simulink model "tqdtqr_rebuild_V3"  (R2021b)
settings: Solver=VariableStepAuto  StartTime=0.0  StopTime=10.0  RelTol=1e-3
undefined symbols (not defined in the file): ATQD_AfterTqMinGain_X_Deg, ATQD_APSCreepBaseTqD_X_kph, ATQD_APSCreepBaseTqD_Y_Deg, ATQD_APSCreepBaseTqR_X_kph, ATQD_APSCreepBaseTqR_Y_Deg, ATQD_APSCreepIterm_X_kph, ATQD_APSCreepIterm_Y_kph, ATQD_APSCreepPterm_X_kph, ATQD_APSCreepPterm_Y_kph, ATQD_APSDecReq_X_kph, ATQD_APSDecReq_Y_mps2, ATQD_APSDecReqCMD_X_kph, ATQD_APSDecReqTs_X_pct, ATQD_APSDecTimeGain_X_Deg, ATQD_APSDecTimeGain_Y_s, ATQD_APSReqLowSpd_X_Deg, ATQD_AutoHoldReleaseBPS_X_Deg, ATQD_AWDLoadTrqnsGain_X_kg, ATQD_AWDLoadTrqnsGain_Y_pct, ATQD_BOSEnBPSPosn_X_kph, ATQD_BOSMap_X_rpm, ATQD_BOSMap_Y_pct, ATQD_CreepBaseTqD_X_kph, ATQD_CreepBaseTqD_Y_Deg, ATQD_CreepBaseTqR_X_kph, ATQD_CreepBaseTqR_Y_Deg, ATQD_CreepBPSDisPosn_X_Deg, ATQD_CreepBPSDisPosnR_X_Deg, ATQD_CreepBPSEnPosn_X_Deg, ATQD_CreepBPSEnPosnR_X_Deg, ATQD_CreepDeltaTq_X_kph, ATQD_CreepIterm_X_kph, ATQD_CreepIterm_Y_kph, ATQD_CreepItermMaxLimit_X_pct, ATQD_CreepPreloadTime_X_kph, ATQD_CreepPreloadTq_X_kph, ATQD_CreepPreloadTq_Y_s, ATQD_CreepProtTq_X_Deg, ATQD_CreepPterm_X_kph, ATQD_CreepPterm_Y_kph, ATQD_CreepRrTqSpRat_X_rpm, ATQD_CreepRrTqSpRat_Y_Nm, ATQD_CreepTargetSpdD_X_pct, ATQD_CreepTargetSpdR_X_pct, ATQD_CreepUpLimitTq_X_rpm, ATQD_DecIneOPDHoldEnDelay_X_Deg, ATQD_DecIneOPDHoldEnDelay_Y_bar, ATQD_ECOTqMapD_X_rpm, ATQD_ECOTqMapD_Y_pct, ATQD_EMTqMapD_X_rpm, ATQD_EMTqMapD_Y_pct, ATQD_EOPDTqMapDCon_X_rpm, ATQD_EOPDTqMapDCon_Y_Deg, ATQD_EstInitVehWeight_X_c, ATQD_FAfterTqCMDGain_X_rpm, ATQD_FAfterTqCMDGain_Y_pct, ATQD_ForceLowSpd_X_Deg, ATQD_ForcePLimitSpd_X_Deg, ATQD_FrLossMAPLowV_X_rpm, ATQD_FrLossMAPLowV_Y_Nm ... (+949)
libraries: simulink x235, hcu_lib x208, tqr x63, tqd x6
(part 12 of 37)

== system tqdtqr_rebuild_V3/Input_Convert/Signal function/MCU Damping Disable Judgement ==
  note: Front / Rear final damping disable flag with vehicle type
  note: Damping disable requested by APS / vehicle speed
  note: Front/Rear MCU damping disable flag
  BSCPIn_outputs : Inport
  BSignalConvert_outputs : Inport  Port=2
  AND2 : Logic  Operator=OR  AllPortsSameDT=off  OutDataTypeStr=boolean
  AND9 : Logic  Operator=OR  AllPortsSameDT=off  OutDataTypeStr=boolean
  Bus Selector : BusSelector  OutputSignals=VVMC_ADASActive_flg,VINP_FrRBCActive_flg,VINP_FrntAxlTrqReqBrk_Nm,VVMC_ACCRequiredAccel_mps2,VINP_RrRBCActive_flg,VINP_RearAxlTrqReqBrk_Nm,VINP_VehSpeed_kph,VTQD_ActAPSPosn_pct,VPMM_DrivetrainSelect_enum
  Bus Selector1 : BusSelector  OutputSignals=VTQD_SCPFrEDURealTMTq_Nm,VTQD_SCPRrEDURealTMTq_Nm
  Constant24 : Constant  Value=KTQD_MCUDmEnFrBrkTq_Nm
  Constant25 : Constant  Value=KTQD_MCUDmEnAccCMD_mps2
  Constant27 : Constant  Value=KTQD_MCUDmEnRrBrkTq_Nm
  Constant40 : Constant  Value=KTQD_ActvDmpDisabAPSPosn_pct  OutDataTypeStr=Inherit: Inherit via back propagation
  Constant41 : Constant  Value=KTQD_ActvDmpDisabVehSpd_kph  OutDataTypeStr=Inherit: Inherit via back propagation
  Constant44 : Constant  Value=KTQD_MCUDmEnAccCMD_mps2
  Constant48 : Constant  Value=ENUM_DRIVETRAIN_FWD
  Constant49 : Constant  Value=ENUM_DRIVETRAIN_AWD
  Constant59 : Constant  Value=ENUM_DRIVETRAIN_RWD
  Constant60 : Constant  Value=ENUM_DRIVETRAIN_AWD
  Constant61 : Constant  Value=FALSE
  Constant62 : Constant  Value=FALSE
  Constant63 : Constant  Value=KTQD_RrDmpDisabReq_flg_ovrdval  OutDataTypeStr=Inherit: Inherit via back propagation
  Constant64 : Constant  Value=KTQD_FrDmpDisabReq_flg_ovrdval  OutDataTypeStr=Inherit: Inherit via back propagation
  Constant65 : Constant  Value=KTQD_MCUDmEnRrBrkTq_Nm
  Constant67 : Constant  Value=KTQD_FrDmpDisabReq_flg_ovrdflg  OutDataTypeStr=Inherit: Inherit via back propagation
  Constant68 : Constant  Value=KTQD_RrDmpDisabReq_flg_ovrdflg  OutDataTypeStr=Inherit: Inherit via back propagation
  Constant9 : Constant  Value=KTQD_MCUDmEnFrBrkTq_Nm
  Data Type Conversion : DataTypeConversion  OutDataTypeStr=boolean
  Data Type Conversion1 : DataTypeConversion  OutDataTypeStr=boolean
  Equal{17..19,23} (4 alike) : RelationalOperator  Operator===  OutDataTypeStr=boolean  RndMeth=Simplest
  Equal{24..25,27..28} (4 alike) : RelationalOperator  OutDataTypeStr=boolean  RndMeth=Simplest
  Equal26 : RelationalOperator  Operator=>  OutDataTypeStr=boolean  RndMeth=Simplest
  Equal29 : RelationalOperator  Operator=>  OutDataTypeStr=boolean  RndMeth=Simplest
  Less Than : RelationalOperator  Operator=<=  OutDataTypeStr=boolean  RndMeth=Simplest
  Less Than1 : RelationalOperator  Operator=<=  OutDataTypeStr=boolean  RndMeth=Simplest
  LiuzgSwitch{16..17,19..20} (4 alike) : Switch  Criteria=u2 ~= 0
      settings: AttributesFormatString=<%<Criteria>>
  Logical Operator{7,10,12..13,15,17..18} (7 alike) : Logic  AllPortsSameDT=off  OutDataTypeStr=boolean
  Logical Operator11 : Logic  Operator=OR  Inputs=3  AllPortsSameDT=off  OutDataTypeStr=boolean
  Logical Operator14 : Logic  Operator=OR  Inputs=3  AllPortsSameDT=off  OutDataTypeStr=boolean
  Logical Operator16 : Logic  Operator=NOT  AllPortsSameDT=off  OutDataTypeStr=boolean
  Logical Operator19 : Logic  Operator=OR  AllPortsSameDT=off  OutDataTypeStr=boolean
  Logical Operator8 : Logic  Operator=OR  AllPortsSameDT=off  OutDataTypeStr=boolean
  Logical Operator9 : Logic  Operator=NOT  AllPortsSameDT=off  OutDataTypeStr=boolean
  Relay : Relay  OnSwitchValue=KTQD_FrMCUDmDisSpd_kph  OffSwitchValue=KTQD_FrMCUDmEnSpd_kph
      settings: AttributesFormatString=|
      | ON : %<OffSwitchValue>
      | OFF : %<OnSwitchValue>
  Relay1 : Relay  OnSwitchValue=KTQD_RrMCUDmDisSpd_kph  OffSwitchValue=KTQD_RrMCUDmEnSpd_kph
      settings: AttributesFormatString=|
      | ON : %<OffSwitchValue>
      | OFF : %<OnSwitchValue>
  SR_Latch1 : hcu_lib/Basic_Blocks/SR_Latch
  SR_Latch2 : hcu_lib/Basic_Blocks/SR_Latch
  VTQD_FrActvDmpDisabReq_flg : Outport
  VTQD_RrActvDmpDisabReq_flg : Outport  Port=2
  wires:
  [VTQD_ActAPSPosn_pct] -> Less Than/1
  LiuzgSwitch17/1 -> LiuzgSwitch20/3
  [VPMM_DrivetrainSelect_enum] -> Equal17/1
  AND2/1 -> LiuzgSwitch16/2
  Logical Operator8/1 -> LiuzgSwitch17/1
  Equal26/1 -> Logical Operator11/3
  [VINP_VehSpeed_kph] -> Relay1/1
  [VINP_FrntAxlTrqReqBrk_Nm] -> Equal24/1
  Constant59/1 -> Equal17/2
  Less Than/1 -> Logical Operator7/1
  Constant61/1 -> LiuzgSwitch16/3
  LiuzgSwitch20/1 -> [VTQD_RrActvDmpDisabReq_flg]  "VTQD_RrActvDmpDisabReq_flg"
  Relay/1 -> Data Type Conversion/1
  [VVMC_ADASActive_flg] -> Logical Operator15/1
  Data Type Conversion/1 -> Logical Operator17/1  "VTQD_FrMCUDmDisSpd_flg"
  Equal24/1 -> Logical Operator10/1
  LiuzgSwitch19/1 -> [VTQD_FrActvDmpDisabReq_flg]  "VTQD_FrActvDmpDisabReq_flg"
  [VTQD_FrADASRegMCUDmDis_flg] -> Logical Operator19/1
  Constant62/1 -> LiuzgSwitch17/3
  Constant41/1 -> Less Than1/2
  [VTQD_RrADASRegMCUDmDis_flg] -> Logical Operator8/1
  Equal18/1 -> AND2/1
  AND9/1 -> LiuzgSwitch17/2
  Constant64/1 -> LiuzgSwitch19/1
  SR_Latch1/1 -> Logical Operator17/2
  [VINP_FrRBCActive_flg] -> Logical Operator12/2
  Data Type Conversion1/1 -> Logical Operator18/1  "VTQD_RrMCUDmDisSpd_flg"
  Constant9/1 -> Equal24/2
  Constant24/1 -> Equal25/2
  Logical Operator14/1 -> SR_Latch2/2
  Constant67/1 -> LiuzgSwitch19/2
  Less Than1/1 -> Logical Operator7/2
  [VINP_FrRBCActive_flg] -> Logical Operator9/1
  [VTQD_SCPFrEDURealTMTq_Nm] -> Equal25/1
  [VVMC_ACCRequiredAccel_mps2] -> Equal29/1
  [VINP_RrRBCActive_flg] -> Logical Operator16/1
  Logical Operator19/1 -> LiuzgSwitch16/1
  Relay1/1 -> Data Type Conversion1/1
  Equal29/1 -> Logical Operator14/3
  Equal25/1 -> Logical Operator10/2
  Logical Operator12/1 -> SR_Latch1/1
  [VTQD_MCUDmpDisabReq_flg] -> Logical Operator8/2
  Constant68/1 -> LiuzgSwitch20/2
  Constant49/1 -> Equal19/2
  Constant60/1 -> Equal23/2
  Equal23/1 -> AND9/2
  SR_Latch2/1 -> Logical Operator18/2
  [VINP_VehSpeed_kph] -> Relay/1
  Logical Operator10/1 -> Logical Operator11/1
  [VTQD_MCUDmpDisabReq_flg] -> Logical Operator19/2
  [VTQD_SCPRrEDURealTMTq_Nm] -> Equal28/1
  Constant63/1 -> LiuzgSwitch20/1
  Equal28/1 -> Logical Operator13/2
  Constant25/1 -> Equal26/2
  Logical Operator17/1 -> [VTQD_FrADASRegMCUDmDis_flg]  "VTQD_FrADASRegMCUDmDis_flg"
  [VINP_RearAxlTrqReqBrk_Nm] -> Equal27/1
  Constant40/1 -> Less Than/2
  Constant48/1 -> Equal18/2
  Logical Operator7/1 -> [VTQD_MCUDmpDisabReq_flg]  "VTQD_MCUDmpDisabReq_flg"
  Equal19/1 -> AND2/2
  Logical Operator16/1 -> Logical Operator14/2
  [VPMM_DrivetrainSelect_enum] -> Equal19/1
  Equal27/1 -> Logical Operator13/1
  [VVMC_ADASActive_flg] -> Logical Operator12/1
  Logical Operator11/1 -> SR_Latch1/2
  Constant27/1 -> Equal28/2
  Logical Operator13/1 -> Logical Operator14/1
  [VPMM_DrivetrainSelect_enum] -> Equal18/1
  Equal17/1 -> AND9/1
  [VVMC_ACCRequiredAccel_mps2] -> Equal26/1
  Constant65/1 -> Equal27/2
  Logical Operator9/1 -> Logical Operator11/2
  [VPMM_DrivetrainSelect_enum] -> Equal23/1
  Logical Operator18/1 -> [VTQD_RrADASRegMCUDmDis_flg]  "VTQD_RrADASRegMCUDmDis_flg"
  [VINP_VehSpeed_kph] -> Less Than1/1
  Constant44/1 -> Equal29/2
  [VINP_RrRBCActive_flg] -> Logical Operator15/2
  LiuzgSwitch16/1 -> LiuzgSwitch19/3
  Logical Operator15/1 -> SR_Latch2/1
  BSCPIn_outputs/1 -> Bus Selector/1
  Bus Selector/1 -> [VVMC_ADASActive_flg]  "<VVMC_ADASActive_flg>"
  Bus Selector/2 -> [VINP_FrRBCActive_flg]  "<VINP_FrRBCActive_flg>"
  Bus Selector/3 -> [VINP_FrntAxlTrqReqBrk_Nm]  "<VINP_FrntAxlTrqReqBrk_Nm>"
  BSignalConvert_outputs/1 -> Bus Selector1/1
  Bus Selector1/1 -> [VTQD_SCPFrEDURealTMTq_Nm]  "<VTQD_SCPFrEDURealTMTq_Nm>"
  Bus Selector/4 -> [VVMC_ACCRequiredAccel_mps2]  "<VVMC_ACCRequiredAccel_mps2>"
  Bus Selector/5 -> [VINP_RrRBCActive_flg]  "<VINP_RrRBCActive_flg>"
  Bus Selector/6 -> [VINP_RearAxlTrqReqBrk_Nm]  "<VINP_RearAxlTrqReqBrk_Nm>"
  Bus Selector/7 -> [VINP_VehSpeed_kph]  "<VINP_VehSpeed_kph>"
  Bus Selector1/2 -> [VTQD_SCPRrEDURealTMTq_Nm]  "<VTQD_SCPRrEDURealTMTq_Nm>"
  Bus Selector/8 -> [VTQD_ActAPSPosn_pct]  "<VTQD_ActAPSPosn_pct>"
  Bus Selector/9 -> [VPMM_DrivetrainSelect_enum]  "<VPMM_DrivetrainSelect_enum>"
  [VTQD_RrActvDmpDisabReq_flg] -> VTQD_RrActvDmpDisabReq_flg/1
  [VTQD_FrActvDmpDisabReq_flg] -> VTQD_FrActvDmpDisabReq_flg/1

== system tqdtqr_rebuild_V3/Input_Convert/Signal function/New Wheel Slide Rate ==
  note: Get vehicle speed base
  note: Get max and min slide rate
  note: Calculate left front wheel slide rate
  note: Calculate right front wheel slide rate
  note: Calculate right rear wheel slide rate
  note: Compare front rear slide rate percent
  note: Calculate left rear wheel slide rate
  note: Compare left right slide rate percent
  BSCPIn_outputs : Inport
  BMain_outputs : Inport  Port=2
  Abs{,1..7} (8 alike) : Abs
  Add : Sum
  Add{1..4} (4 alike) : Sum  Inputs=+-
  Bus Selector : BusSelector  OutputSignals=task_time_s,VINP_RRRawWhlSpeed_kph,VINP_RFRawWhlSpeed_kph,VINP_LRRawWhlSpeed_kph,VINP_LFRawWhlSpeed_kph,VINP_VehSpeed_kph
  Bus Selector1 : BusSelector  OutputSignals=VTQR_NoABSREDUWhlTqReq_Nm,VTQR_NoABSFEDUWhlTqReq_Nm
  Constant{1,4,6,9,11,15,18,135} (8 alike) : Constant  Value=eps
  Constant{5,10,14,128} (4 alike) : Constant  Value=KTQD_NewSlideRateTs_c
  Constant{2,7,12,16,19} (5 alike) : Constant  Value=ZERO_FLOAT
  Constant{3,8,13,17} (4 alike) : Constant  Value=ONE_PERCENT
  Data Type Conversion{,1..3} (4 alike) : DataTypeConversion  OutDataTypeStr=single
  Delay : Delay  DelayLength=1  InitialCondition=single(0.0)
      settings: AttributesFormatString=%<InitialCondition>
  Delay1 : Delay  DelayLength=1  InitialCondition=single(0.0)
      settings: AttributesFormatString=%<InitialCondition>
  Divide{,1..7} (8 alike) : Product  Inputs=*/
  FirstOrderFilter{,1..3} (4 alike) : hcu_lib/Basic_Blocks/FirstOrderFilter
  Max{,1..3} (4 alike) : MinMax  Function=max  Inputs=2
  Max4 : MinMax  Function=max  Inputs=4
  Max5 : MinMax  Inputs=4
  Min : MinMax  Inputs=5
  Relational Operator{,1..3} (4 alike) : RelationalOperator  Operator=<=  OutDataTypeStr=boolean  RndMeth=Simplest
  Relational Operator{4..7} (4 alike) : RelationalOperator  OutDataTypeStr=boolean  RndMeth=Simplest
  Relational Operator8 : RelationalOperator  Operator=>  OutDataTypeStr=boolean  RndMeth=Simplest
  Switch{,1..8} (9 alike) : Switch  Criteria=u2 ~= 0
      settings: AttributesFormatString=%<Criteria>
  VTQD_MaxWhlSlideRate_pct : Outport
  VTQD_MinWhlSlideRate_pct : Outport  Port=2
  VTQD_LeftSlideRate_pct : Outport  Port=3
  VTQD_RightSlideRate_pct : Outport  Port=4
  VTQD_FrontSlideRate_pct : Outport  Port=5
  VTQD_RearSlideRate_pct : Outport  Port=6
  VTQD_LFSlideRate_pct : Outport  Port=7
  VTQD_LRSlideRate_pct : Outport  Port=8
  VTQD_RFSlideRate_pct : Outport  Port=9
  VTQD_RRSlideRate_pct : Outport  Port=10
  wires:
  BSCPIn_outputs/1 -> Bus Selector/1
  Bus Selector/1 -> [task_time_s]  "<task_time_s>"
  Bus Selector/3 -> [VINP_RFRawWhlSpeed_kph]  "<VINP_RFRawWhlSpeed_kph>"
  Bus Selector/2 -> [VINP_RRRawWhlSpeed_kph]  "<VINP_RRRawWhlSpeed_kph>"
  Bus Selector/6 -> [VINP_VehSpeed_kph]  "<VINP_VehSpeed_kph>"
  Bus Selector/5 -> [VINP_LFRawWhlSpeed_kph]  "<VINP_LFRawWhlSpeed_kph>"
  Bus Selector/4 -> [VINP_LRRawWhlSpeed_kph]  "<VINP_LRRawWhlSpeed_kph>"
  [VTQD_MaxWhlSlideRate_pct] -> VTQD_MaxWhlSlideRate_pct/1
  [VTQD_MinWhlSlideRate_pct] -> VTQD_MinWhlSlideRate_pct/1
  [VTQD_LeftSlideRate_pct] -> VTQD_LeftSlideRate_pct/1
  [VTQD_RightSlideRate_pct] -> VTQD_RightSlideRate_pct/1
  [VTQD_FrontSlideRate_pct] -> VTQD_FrontSlideRate_pct/1
  [VTQD_RearSlideRate_pct] -> VTQD_RearSlideRate_pct/1
  [VTQD_LFSlideRate_pct] -> VTQD_LFSlideRate_pct/1
  [VTQD_LRSlideRate_pct] -> VTQD_LRSlideRate_pct/1
  [VTQD_RFSlideRate_pct] -> VTQD_RFSlideRate_pct/1
  [VTQD_RRSlideRate_pct] -> VTQD_RRSlideRate_pct/1
  Abs3/1 -> Relational Operator5/2
  [VTQR_NoABSFEDUWhlTqReq_Nm] -> Delay/1
  Constant11/1 -> Data Type Conversion/1
  [VTQD_VehSpeed4Cal_kph] -> Max1/1
  Data Type Conversion/1 -> Max2/2
  Constant6/1 -> Data Type Conversion1/1
  Data Type Conversion1/1 -> Max1/2
  Data Type Conversion2/1 -> Max/2
  Abs2/1 -> Relational Operator5/1
  Divide5/1 -> Switch2/3
  Constant15/1 -> Data Type Conversion3/1
  Constant135/1 -> Data Type Conversion2/1
  Data Type Conversion3/1 -> Max3/2
  FirstOrderFilter1/1 -> Divide2/1
  Switch6/1 -> [VTQD_FrontSlideRate_pct]  "VTQD_FrontSlideRate_pct"
  [VTQD_VehSpeed4Cal_kph] -> Add3/2
  Switch/1 -> FirstOrderFilter/1
  Add3/1 -> Divide5/1
  [VTQD_VehSpeed4Cal_kph] -> Max3/1
  [VTQD_VehSpeed4Cal_kph] -> Max2/1
  Max2/1 -> Divide5/2
  [VTQD_LRSlideRate_pct] -> Abs1/1
  [VINP_RRRawWhlSpeed_kph] -> Add4/1
  FirstOrderFilter/1 -> Divide/1
  Abs1/1 -> Relational Operator4/2
  [VTQD_RFSlideRate_pct] -> Max4/3
  Constant1/1 -> Relational Operator/2
  Abs5/1 -> Relational Operator6/2
  Relational Operator/1 -> Switch/2
  [VTQD_VehSpeed4Cal_kph] -> Max/1
  Constant4/1 -> Relational Operator1/2
  [task_time_s] -> FirstOrderFilter3/2
  [VTQD_VehSpeed4Cal_kph] -> Add4/2
  [VTQD_RFSlideRate_pct] -> Switch6/3
  [task_time_s] -> FirstOrderFilter2/2
  [VTQD_RRSlideRate_pct] -> Abs3/1
  Constant5/1 -> FirstOrderFilter1/3
  Add/1 -> Relational Operator8/1
  [VTQD_VehSpeed4Cal_kph] -> Add1/2
  [VTQD_LFSlideRate_pct] -> Switch6/1
  [VINP_VehSpeed_kph] -> Min/5
  FirstOrderFilter3/1 -> Divide6/1
  Abs7/1 -> Relational Operator7/2
  Divide6/1 -> [VTQD_RRSlideRate_pct]  "VTQD_RRSlideRate_pct"
  [VTQR_NoABSREDUWhlTqReq_Nm] -> Delay1/1
  [VINP_VehSpeed_kph] -> Switch8/3
  [VINP_LRRawWhlSpeed_kph] -> Min/2
  Relational Operator5/1 -> Switch5/2
  Abs/1 -> Relational Operator4/1
  [VINP_RRRawWhlSpeed_kph] -> Min/4
  [VTQD_VehSpeed4Cal_kph] -> Relational Operator3/1
  Max5/1 -> [VTQD_MinWhlSlideRate_pct]  "VTQD_MinWhlSlideRate_pct"
  [VINP_LFRawWhlSpeed_kph] -> Min/1
  [VTQD_LFSlideRate_pct] -> Max4/1
  Switch8/1 -> [VTQD_VehSpeed4Cal_kph]  "VTQD_VehSpeed4Cal_kph"
  [VTQD_RRSlideRate_pct] -> Switch5/3
  Add2/1 -> Divide1/1
  Delay/1 -> Add/1
  Divide4/1 -> [VTQD_RFSlideRate_pct]  "VTQD_RFSlideRate_pct"
  [VTQD_VehSpeed4Cal_kph] -> Relational Operator1/1
  Constant19/1 -> Relational Operator8/2
  [VTQD_RFSlideRate_pct] -> Abs5/1
  Relational Operator8/1 -> Switch8/2
  Abs4/1 -> Relational Operator6/1
  [VINP_RFRawWhlSpeed_kph] -> Min/3
  Constant13/1 -> Divide4/2
  Max/1 -> Divide1/2
  [VTQD_LFSlideRate_pct] -> Abs4/1
  Switch4/1 -> [VTQD_LeftSlideRate_pct]  "VTQD_LeftSlideRate_pct"
  Divide3/1 -> Switch1/3
  Constant10/1 -> FirstOrderFilter2/3
  Constant17/1 -> Divide6/2
  Relational Operator1/1 -> Switch1/2
  Relational Operator4/1 -> Switch4/2
  Constant7/1 -> Switch1/1
  [VTQD_LRSlideRate_pct] -> Max4/2
  Divide2/1 -> [VTQD_LRSlideRate_pct]  "VTQD_LRSlideRate_pct"
  Relational Operator2/1 -> Switch2/2
  Min/1 -> Switch8/1
  [VTQD_RFSlideRate_pct] -> Abs2/1
  Max1/1 -> Divide3/2
  [VINP_LRRawWhlSpeed_kph] -> Add1/1
  [VTQD_RFSlideRate_pct] -> Switch5/1
  Max4/1 -> [VTQD_MaxWhlSlideRate_pct]  "VTQD_MaxWhlSlideRate_pct"
  [VTQD_RRSlideRate_pct] -> Max5/4
  Constant128/1 -> FirstOrderFilter/3
  Add4/1 -> Divide7/1
  [VTQD_LFSlideRate_pct] -> Switch4/1
  [VTQD_LRSlideRate_pct] -> Max5/2
  [VTQD_LRSlideRate_pct] -> Switch4/3
  Add1/1 -> Divide3/1
  Constant12/1 -> Switch2/1
  Divide1/1 -> Switch/3
  Constant2/1 -> Switch/1
  [VTQD_VehSpeed4Cal_kph] -> Add2/2
  [VTQD_VehSpeed4Cal_kph] -> Relational Operator/1
  [VTQD_RRSlideRate_pct] -> Abs7/1
  [VTQD_RFSlideRate_pct] -> Max5/3
  [VTQD_RRSlideRate_pct] -> Max4/4
  Constant3/1 -> Divide/2
  [VINP_LFRawWhlSpeed_kph] -> Add2/1
  [task_time_s] -> FirstOrderFilter/2
  [VTQD_VehSpeed4Cal_kph] -> Relational Operator2/1
  [VTQD_LRSlideRate_pct] -> Switch7/1
  Divide7/1 -> Switch3/3
  Max3/1 -> Divide7/2
  Delay1/1 -> Add/2
  Switch7/1 -> [VTQD_RearSlideRate_pct]  "VTQD_RearSlideRate_pct"
  [VTQD_LFSlideRate_pct] -> Max5/1
  Relational Operator3/1 -> Switch3/2
  FirstOrderFilter2/1 -> Divide4/1
  Divide/1 -> [VTQD_LFSlideRate_pct]  "VTQD_LFSlideRate_pct"
  Relational Operator7/1 -> Switch7/2
  Abs6/1 -> Relational Operator7/1
  Constant18/1 -> Relational Operator3/2
  [VTQD_RRSlideRate_pct] -> Switch7/3
  Constant14/1 -> FirstOrderFilter3/3
  [VINP_RFRawWhlSpeed_kph] -> Add3/1
  Constant16/1 -> Switch3/1
  Switch5/1 -> [VTQD_RightSlideRate_pct]  "VTQD_RightSlideRate_pct"
  [task_time_s] -> FirstOrderFilter1/2
  Switch1/1 -> FirstOrderFilter1/1
  Constant9/1 -> Relational Operator2/2
  Constant8/1 -> Divide2/2
  Switch3/1 -> FirstOrderFilter3/1
  [VTQD_LFSlideRate_pct] -> Abs/1
  Relational Operator6/1 -> Switch6/2
  Switch2/1 -> FirstOrderFilter2/1
  [VTQD_LRSlideRate_pct] -> Abs6/1
  BMain_outputs/1 -> Bus Selector1/1
  Bus Selector1/1 -> [VTQR_NoABSREDUWhlTqReq_Nm]  "<VTQR_NoABSREDUWhlTqReq_Nm>"
  Bus Selector1/2 -> [VTQR_NoABSFEDUWhlTqReq_Nm]  "<VTQR_NoABSFEDUWhlTqReq_Nm>"

== system tqdtqr_rebuild_V3/Input_Convert/Signal function/OPD Hold ==
  BSCPIn_outputs : Inport
  BSignalConvert_outputs : Inport  Port=2
  DriverWhlTqDemFunc_outputs : Inport  Port=3
  BMain_outputs : Inport  Port=4
  VTQD_GearActualPosn_enum : Inport  Port=5
  VTQD_ActWhlSkipSta_enum : Inport  Port=6
  VTQD_SkipDirect_enum : Inport  Port=7
  VTQD_ParkRequest_flg : Inport  Port=8
  VTQD_ForceP_flg : Inport  Port=9
  VTQD_EPBCarWashMode_flg : Inport  Port=10
  Bus Selector : BusSelector  OutputSignals=task_time_s,VINP_EPBSta_enum,VVMC_ADASActive_flg,VPMM_PowerSta_enum,VVMC_CruzActive_flg,VVMC_EstSlope_Deg,VINP_FrPTCSActive_flg,VINP_RrPTCSActive_flg,VINP_ESCActive_flg,VINP_ABSActive_flg,VVMC_APSActive_flg,VTQD_ActBPSPosn_pct,VTQD_LimpHomeAct_flg,VVMC_LongAcc_Gps,VTQD_ActAPSPosn_pct,VINP_DrDoorSW_flg,VPMM_DrSeatSta_enum,VTQD_ShifterHandleCmd_enum,VINP_BrkSwSta_flg,VINP_DriverSeatBeltCmd_flg,VINP_MCPressure_bar
  Bus Selector1 : BusSelector  OutputSignals=VTQD_RegenMode_enum,VTQD_VehActSpd_kph,VTQD_LowIdleAccPedal_flg,VTQD_TqTargetShaftSpd_rpm
  Bus Selector2 : BusSelector  OutputSignals=VTQR_NoABSFEDUWhlTqReq_Nm,VTQR_NoABSREDUWhlTqReq_Nm
  Bus Selector3 : BusSelector  OutputSignals=VTQD_PedAccTqEn_flg,VTQD_IVIRockModeEn_flg
  Constant34 : Constant  Value=KTQD_IVICreepOnSW_flg
  Deceleration Calculation : Subsystem
  "OPDHold Request " : Subsystem
  Parking Requeest Backup : Subsystem  AncestorBlock=tqd/TQD/TorqueDemand/TorqueModule/OPD Hold/Parking Requeest Backup
  Release Condition : Subsystem
  System Status : Subsystem
  VTQD_APSStaSys_enum : Outport
  VTQD_APSReq_enum : Outport  Port=2
  VTQD_APSDecReqA_flg : Outport  Port=3
  VTQD_APSDecReq_mps2 : Outport  Port=4
  VTQD_ActParkRequest_flg : Outport  Port=5
  VTQD_APSReqTimer_s : Outport  Port=6
  VTQD_OPDHoldEnRel_flg : Outport  Port=7
  VTQD_OPDHoldAllowPark_flg : Outport  Port=8
  VTQD_OPDHoldLamp_flg : Outport  Port=9
  VTQD_OPDHoldActRelTq_Nm : Outport  Port=10
  VTQD_OPDHoldDelayForP_flg : Outport  Port=11
  VTQD_OPDHoldAlarm_flg : Outport  Port=12
  VTQD_OPDHoldForceEn_flg : Outport  Port=13
  wires:
  [VTQD_ActWhlSkipSta_enum] -> System Status/19(VTQD_ActWhlSkipSta_enum)
  [VTQD_LimpHomeAct_flg] -> System Status/21(VTQD_LimpHomeAct_flg)
  [VTQD_PedAccTqEn_flg] -> System Status/16(VTQD_PedAccTqEn_flg)
  [VTQD_SkipDirect_enum] -> System Status/20(VTQD_SkipDirect_enum)
  [task_time_s] -> Release Condition/6(task_time_s)
  [VTQD_APSDecReqA_flg] -> Deceleration Calculation/5(VTQD_APSDecReqA_flg)
  System Status/2(VTQD_OPDHoldDelayForP_flg) -> [VTQD_OPDHoldDelayForP_flg]
  [VTQD_IVIRockModeEn_flg] -> System Status/18(VTQD_IVIRockModeEn_flg)
  [VINP_ABSActive_flg] -> System Status/14(VINP_ABSActive_flg)
  Parking Requeest Backup/2(VTQD_OPDHoldAllowPark_flg) -> [VTQD_OPDHoldAllowPark_flg]
  Deceleration Calculation/1(VTQD_APSDecReq_mps2) -> [VTQD_APSDecReq_mps2]
  "OPDHold Request "/3(VTQD_APSDecReqA_flg) -> [VTQD_APSDecReqA_flg]
  [task_time_s] -> Deceleration Calculation/7(task_time_s)
  [VVMC_EstSlope_Deg] -> Release Condition/1(VVMC_EstSlope_Deg)
  [task_time_s] -> Parking Requeest Backup/4(task_time_s)
  [VTQD_OPDHoldRgnOn2Off_flg] -> Release Condition/9(VTQD_OPDHoldRgnOn2Off_flg)
  System Status/3(VTQD_OPDHoldRgnOn2Off_flg) -> [VTQD_OPDHoldRgnOn2Off_flg]
  [VTQD_AutoHoldRelease_flg] -> System Status/4(VTQD_AutiHoldRelease_flg)
  [VTQD_LowIdleAccPedal_flg] -> Release Condition/8(VTQD_LowIdleAccPedal_flg)
  [VTQD_AutoHoldRelease_flg] -> Deceleration Calculation/6(VTQD_AutiHoldRelease_flg)
  [VTQD_ParkRequest_flg] -> Parking Requeest Backup/3(VTQD_ParkRequest_flg)
  [VVMC_EstSlope_Deg] -> "OPDHold Request "/5(VVMC_EstSlope_Deg)
  [VTQR_NoABSREDUWhlTqReq_Nm] -> Release Condition/4(VTQR_NoABSREDUWhlTqReq_Nm)
  [VTQR_NoABSFEDUWhlTqReq_Nm] -> Release Condition/3(VTQR_NoABSFEDUWhlTqReq_Nm)
  [VVMC_CruzActive_flg] -> System Status/7(VVMC_CruzActive_flg)
  Parking Requeest Backup/1(VTQD_ActParkRequest_flg) -> [VTQD_ActParkRequest_flg]
  [VINP_EPBSta_enum] -> System Status/2(VINP_EPBSta_enum)
  [VTQD_ActBPSPosn_pct] -> Release Condition/5(VTQD_ActBPSPosn_pct)
  [VTQD_AutoHoldRelease_flg] -> Parking Requeest Backup/5(VTQD_AutiHoldRelease_flg)
  [VTQD_RegenMode_enum] -> System Status/3(VTQD_RegenMode_enum)
  [VTQD_GearActualPosn_enum] -> System Status/1(VTQD_GearActualPosn_enum)
  [VVMC_EstSlope_Deg] -> Deceleration Calculation/4(VVMC_EstSlope_Deg)
  [VTQD_APSReqTimer_s] -> Parking Requeest Backup/2(VTQD_APSReqTimer_s)
  [VTQD_APSReqTimer_s] -> Deceleration Calculation/3(VTQD_APSReqTimer_s)
  [VINP_IVICreepOnSW_flg] -> System Status/17(VINP_IVICreepOnSW_flg)
  [VTQD_VehActSpd_kph] -> Deceleration Calculation/1(VTQD_VehActSpd_kph)
  "OPDHold Request "/1(VTQD_APSReqTimer_s) -> [VTQD_APSReqTimer_s]
  [VTQD_AutoHoldRelease_flg] -> "OPDHold Request "/3(VTQD_AutiHoldRelease_flg)
  [VTQD_ActAPSPosn_pct] -> Deceleration Calculation/8(VTQD_ActAPSPosn_pct)
  System Status/1(VTQD_APSStaSys_enum) -> [VTQD_APSStaSys_enum]
  [VTQD_VehActSpd_kph] -> Release Condition/2(VTQD_VehActSpd_kph)
  [VVMC_ADASActive_flg] -> System Status/5(VVMC_ADASActive_flg)
  Release Condition/2(VTQD_OPDHoldEnRel_flg) -> [VTQD_OPDHoldEnRel_flg]
  [VTQD_VehActSpd_kph] -> System Status/8(VTQD_VehActSpd_kph)
  "OPDHold Request "/2(VTQD_APSReq_enum) -> [VTQD_APSReq_enum]
  [VINP_FrPTCSActive_flg] -> System Status/11(VINP_FrPTCSActive_flg)
  [VINP_ESCActive_flg] -> System Status/13(VINP_ESCActive_flg)
  [VINP_RrPTCSActive_flg] -> System Status/12(VINP_RrPTCSActive_flg)
  Release Condition/3(VTQD_OPDHoldActRelTq_Nm) -> [VTQD_OPDHoldActRelTq_Nm]
  [VTQD_APSReqTimer_s] -> Release Condition/7(VTQD_APSReqTimer_s)
  [VTQD_APSReq_enum] -> Parking Requeest Backup/1(VTQD_APSReq_enum)
  [VVMC_EstSlope_Deg] -> System Status/9(VVMC_EstSlope_Deg)
  [VVMC_LongAcc_Gps] -> Deceleration Calculation/2(VVMC_LongAcc_Gps)
  [task_time_s] -> System Status/10(task_time_s)
  [task_time_s] -> "OPDHold Request "/4(task_time_s)
  [VPMM_PwrSta_enum] -> System Status/6(VPMM_PwrSta_enum)
  Release Condition/1(VTQD_AutoHoldRelease_flg) -> [VTQD_AutoHoldRelease_flg]
  [VTQD_APSStaSys_enum] -> "OPDHold Request "/2(VTQD_APSStaSys_enum)
  [VVMC_APSActive_flg] -> System Status/15(VVMC_APSActive_flg)
  "OPDHold Request "/4(VTQD_OPDHoldLamp_flg) -> [VTQD_OPDHoldLamp_flg]
  [VTQD_VehActSpd_kph] -> "OPDHold Request "/1(VTQD_VehActSpd_kph)
  BSCPIn_outputs/1 -> Bus Selector/1
  BSignalConvert_outputs/1 -> Bus Selector1/1
  Bus Selector/2 -> [VINP_EPBSta_enum]  "<VINP_EPBSta_enum>"
  Bus Selector1/1 -> [VTQD_RegenMode_enum]  "<VTQD_RegenMode_enum>"
  Bus Selector/3 -> [VVMC_ADASActive_flg]  "<VVMC_ADASActive_flg>"
  Bus Selector/4 -> [VPMM_PwrSta_enum]  "<VPMM_PowerSta_enum>"
  Bus Selector/5 -> [VVMC_CruzActive_flg]  "<VVMC_CruzActive_flg>"
  Bus Selector1/2 -> [VTQD_VehActSpd_kph]  "<VTQD_VehActSpd_kph>"
  Bus Selector/6 -> [VVMC_EstSlope_Deg]  "<VVMC_EstSlope_Deg>"
  Bus Selector/1 -> [task_time_s]  "<task_time_s>"
  Bus Selector/7 -> [VINP_FrPTCSActive_flg]  "<VINP_FrPTCSActive_flg>"
  Bus Selector/8 -> [VINP_RrPTCSActive_flg]  "<VINP_RrPTCSActive_flg>"
  Bus Selector/9 -> [VINP_ESCActive_flg]  "<VINP_ESCActive_flg>"
  Bus Selector/10 -> [VINP_ABSActive_flg]  "<VINP_ABSActive_flg>"
  Bus Selector/11 -> [VVMC_APSActive_flg]  "<VVMC_APSActive_flg>"
  DriverWhlTqDemFunc_outputs/1 -> Bus Selector3/1
  Bus Selector3/1 -> [VTQD_PedAccTqEn_flg]  "<VTQD_PedAccTqEn_flg>"
  Constant34/1 -> [VINP_IVICreepOnSW_flg]  "VTQD_IVICreepOnSW_flg"
  Bus Selector3/2 -> [VTQD_IVIRockModeEn_flg]  "<VTQD_IVIRockModeEn_flg>"
  Bus Selector/12 -> [VTQD_ActBPSPosn_pct]  "<VTQD_ActBPSPosn_pct>"
  Bus Selector/13 -> [VTQD_LimpHomeAct_flg]  "<VTQD_LimpHomeAct_flg>"
  Bus Selector1/3 -> [VTQD_LowIdleAccPedal_flg]  "<VTQD_LowIdleAccPedal_flg>"
  Bus Selector/14 -> [VVMC_LongAcc_Gps]  "<VVMC_LongAcc_Gps>"
  Bus Selector/15 -> [VTQD_ActAPSPosn_pct]  "<VTQD_ActAPSPosn_pct>"
  [VTQD_APSStaSys_enum] -> VTQD_APSStaSys_enum/1
  [VTQD_APSReq_enum] -> VTQD_APSReq_enum/1
  [VTQD_APSDecReqA_flg] -> VTQD_APSDecReqA_flg/1
  [VTQD_APSDecReq_mps2] -> VTQD_APSDecReq_mps2/1
  [VTQD_ActParkRequest_flg] -> VTQD_ActParkRequest_flg/1
  [VTQD_OPDHoldAllowPark_flg] -> VTQD_OPDHoldAllowPark_flg/1
  [VTQD_OPDHoldLamp_flg] -> VTQD_OPDHoldLamp_flg/1
  [VTQD_OPDHoldActRelTq_Nm] -> VTQD_OPDHoldActRelTq_Nm/1
  [VTQD_OPDHoldDelayForP_flg] -> VTQD_OPDHoldDelayForP_flg/1
  VTQD_GearActualPosn_enum/1 -> [VTQD_GearActualPosn_enum]
  VTQD_ActWhlSkipSta_enum/1 -> [VTQD_ActWhlSkipSta_enum]
  VTQD_SkipDirect_enum/1 -> [VTQD_SkipDirect_enum]
  VTQD_ParkRequest_flg/1 -> [VTQD_ParkRequest_flg]
  [VTQD_APSReqTimer_s] -> VTQD_APSReqTimer_s/1
  [VTQD_OPDHoldEnRel_flg] -> VTQD_OPDHoldEnRel_flg/1
  BMain_outputs/1 -> Bus Selector2/1
  Bus Selector2/1 -> [VTQR_NoABSFEDUWhlTqReq_Nm]  "<VTQR_NoABSFEDUWhlTqReq_Nm>"
  Bus Selector2/2 -> [VTQR_NoABSREDUWhlTqReq_Nm]  "<VTQR_NoABSREDUWhlTqReq_Nm>"
  [VTQD_ForceP_flg] -> System Status/22(VTQD_ForceP_flg)
  [VINP_DrDoorSW_flg] -> System Status/23(VINP_DrDoorSW_flg)
  [VPMM_DrSeatSta_enum] -> System Status/24(VPMM_DrSeatSta_enum)
  [VTQD_EPBCarWashMode_flg] -> System Status/25(VTQD_EPBCarWashMode_flg)
  [VINP_ShifterHandleCmd_enum] -> System Status/26(VINP_ShifterHandleCmd_enum)
  [VTQD_BrkSwSta_flg] -> System Status/27(VTQD_BrkSwSta_flg)
  [VTQD_TqTargetShaftSpd_rpm] -> System Status/28(VTQD_TqTargetShaftSpd_rpm)
  [VINP_DriverSeatBeltCmd_flg] -> System Status/29(VINP_DriverSeatBeltCmd_flg)
  [VINP_MCPressure_bar] -> System Status/30(VINP_MCPressure_bar)
  VTQD_ForceP_flg/1 -> [VTQD_ForceP_flg]
  Bus Selector/16 -> [VINP_DrDoorSW_flg]  "<VINP_DrDoorSW_flg>"
  Bus Selector/17 -> [VPMM_DrSeatSta_enum]  "<VPMM_DrSeatSta_enum>"
  VTQD_EPBCarWashMode_flg/1 -> [VTQD_EPBCarWashMode_flg]
  Bus Selector/18 -> [VINP_ShifterHandleCmd_enum]  "<VTQD_ShifterHandleCmd_enum>"
  Bus Selector/19 -> [VTQD_BrkSwSta_flg]  "<VINP_BrkSwSta_flg>"
  Bus Selector1/4 -> [VTQD_TqTargetShaftSpd_rpm]  "<VTQD_TqTargetShaftSpd_rpm>"
  Bus Selector/20 -> [VINP_DriverSeatBeltCmd_flg]  "<VINP_DriverSeatBeltCmd_flg>"
  Bus Selector/21 -> [VINP_MCPressure_bar]  "<VINP_MCPressure_bar>"
  System Status/4(VTQD_OPDHoldForceEn_flg) -> [VTQD_OPDHoldForceEn_flg]
  [VTQD_OPDHoldForceEn_flg] -> "OPDHold Request "/6(VTQD_OPDHoldForceEn_flg)
  "OPDHold Request "/5(VTQD_OPDHoldAlarm_flg) -> [VTQD_OPDHoldAlarm_flg]
  [VTQD_OPDHoldForceEn_flg] -> Deceleration Calculation/10(VTQD_OPDHoldForceEn_flg)
  [VTQD_LowIdleAccPedal_flg] -> Deceleration Calculation/9(VTQD_LowIdleAccPedal_flg)
  [VTQD_OPDHoldAlarm_flg] -> VTQD_OPDHoldAlarm_flg/1
  [VTQD_OPDHoldForceEn_flg] -> VTQD_OPDHoldForceEn_flg/1

== system tqdtqr_rebuild_V3/Input_Convert/Signal function/Regen level define ==
  note: Regen LV calculate
  note: Trailer mode define / OPD mode disable flag
  note: One pedal mode disable condition
  note: Check BCM personalized settings -> flash data / user settings
  note: BCM user identified check flag
  note: Regen up down signal
  note: Regen up down button determine
  BSCPIn_outputs : Inport
  BSignalConvert_outputs : Inport  Port=2
  VTQD_LFSlideRate_pct : Inport  Port=3
  VTQD_RFSlideRate_pct : Inport  Port=4
  VTQD_LRSlideRate_pct : Inport  Port=5
  VTQD_RRSlideRate_pct : Inport  Port=6
  VTQD_GearActualPosn_enum : Inport  Port=7
  VTQD_DOALatchReq_flg : Inport  Port=8
  " " : Constant  Value=KTQD_RegenMode_enum_ovrdval
  "  " : Constant  Value=KTQD_RegenMode_enum_ovrdflg
  AND10 : Logic  AllPortsSameDT=off  OutDataTypeStr=boolean
  AND11 : Logic  AllPortsSameDT=off  OutDataTypeStr=boolean
  AND23 : Logic  AllPortsSameDT=off  OutDataTypeStr=boolean
  AND24 : Logic  Inputs=8  AllPortsSameDT=off  OutDataTypeStr=boolean
  AND8 : Logic  Inputs=3  AllPortsSameDT=off  OutDataTypeStr=boolean
  Abs3 : Abs
  Abs4 : Abs
  Add1 : Sum  Inputs=+-
  Add2 : Sum  Inputs=+-
  Bus Selector : BusSelector  OutputSignals=task_time_s,VINP_FlashRegenMode_enum,VPMM_PowerSta_enum,VINP_ADASACCSta_enum,VVMC_CCCtrlSta_enum,VBCM_BrakeLamp_flg,VINP_VehSpeed_kph,VINP_SmartEcoModeSW_flg,VINP_IVISnowModeCmd_flg,VBCM_UserNow_enum,VINP_IVITrailerModeSWSta_flg,VINP_VehicleType_enum,VBCM_RegenModeUserSetting_enum,VPMM_SysPowerMode_enum,VINP_DIDNVHPedalLim_flg
  Bus Selector2 : BusSelector  OutputSignals=VTQD_RegenMode_enum,VTQD_SCPSWCRegenUp_flg,VTQD_SCPSWCRegenDown_flg
  Constant1 : Constant  Value=ENUM_PWRSTASW_ON
  Constant{99..100,114..115} (4 alike) : Constant  Value=FALSE
  Constant101 : Constant  Value=KTQD_RegenModeMemo_flg
  Constant102 : Constant  Value=KTQD_DefaultRegenMode_enum
  Constant110 : Constant  Value=KTQD_OPDDisSlideRateDT_s
  Constant111 : Constant  Value=ENUM_GEARACTUALPOSN_P
  Constant112 : Constant  Value=ENUM_VEHICLETYPE_D31HAWD
  Constant113 : Constant  Value=ENUM_VEHICLETYPE_D31HRWD
  Constant116 : Constant  Value=ENUM_VEHICLETYPE_D31HAWD
  Constant117 : Constant  Value=ENUM_VEHICLETYPE_D31HRWD
  Constant118 : Constant  Value=ENUM_VEHICLETYPE_P71
  Constant119 : Constant  Value=KTQD_NVHPedLimRegen_enum
  Constant120 : Constant  Value=KTQD_NVHPedLimRegen_enum
  Constant135 : Constant  Value=KTQD_TrailerModeSW_flg_ovrdflg
  Constant136 : Constant  Value=KTQD_TrailerModeSW_flg_ovrdval
  Constant137 : Constant  Value=ENUM_REGENSWSTA_LONGPRESSUP
  Constant138 : Constant  Value=ENUM_POWERSTA_ON
  Constant139 : Constant  Value=ENUM_POWERSTA_READY
  Constant140 : Constant  Value=ENUM_BCMUSERNOWSET_INVALID
  Constant141 : Constant  Value=ENUM_BCMUSERNOWSET_GUEST
  Constant142 : Constant  Value=ENUM_BCMUSERNOWSET_RENT
  Constant143 : Constant  Value=ENUM_RGNMODEUSERSET_OFF
  Constant144 : Constant  Value=ENUM_RGNMODEUSERSET_INVALID
  Constant2 : Constant  Value=ENUM_REGENLEVEL_OFF
  Constant3 : Constant  Value=ENUM_REGENLEVEL_OPD
  Constant4 : Constant  Value=KTQD_DOAOPDReqSW_flg
  Constant87 : Constant  Value=KTQD_RegenMode_enum_ovrdflg
  Constant88 : Constant  Value=KTQD_RegenMode_enum_ovrdval
  Constant91 : Constant  Value=ENUM_VEHICLETYPE_P71
  Constant92 : Constant  Value=KTQD_OPDDisSlideRateDev_pct
  Constant94 : Constant  Value=KTQD_OutSideTemp_C
  Constant95 : Constant  Value=ENUM_REGENLEVEL_OPD
  Data Type Conversion7 : DataTypeConversion  OutDataTypeStr=boolean
  Delay{1,5,7,9} (4 alike) : Delay  DelayLength=1  InitialCondition=ENUM_REGENLEVEL_OFF
      settings: AttributesFormatString=%<InitialCondition>
  Delay6 : Delay  DelayLength=1  InitialCondition=uint8(0)
      settings: AttributesFormatString=%<InitialCondition>
  DelayEnable : hcu_lib/Basic_Blocks/DelayEnable
  Detect Change1 : simulink/Logic and Bit Operations/Detect Change  vinit=boolean(0)  OutDataTypeStr=boolean
  Detect Change3 : simulink/Logic and Bit Operations/Detect Change  vinit=boolean(0)  OutDataTypeStr=boolean
  Detect Increase : simulink/Logic and Bit Operations/Detect Increase  vinit=boolean(0)  OutDataTypeStr=boolean
  Detect Increase1 : simulink/Logic and Bit Operations/Detect Increase  vinit=boolean(0)  OutDataTypeStr=boolean
  Equal{1,41..42,46..48,54..55,59..60} (10 alike) : RelationalOperator  Operator===  OutDataTypeStr=boolean  RndMeth=Simplest
  Equal{2,43..45,56..58} (7 alike) : RelationalOperator  Operator=~=  OutDataTypeStr=boolean  RndMeth=Simplest
  KTQD_ICERoadDisTemp_C KTQD_ICERoadTemp_C : Relay  OnSwitchValue=KTQD_ICERoadDisTemp_C  OffSwitchValue=KTQD_ICERoadTemp_C  OutDataTypeStr=boolean
  Latch : hcu_lib/Basic_Blocks/Latch
  Max1 : MinMax  Function=max  Inputs=2
  NOT1 : Logic  Operator=NOT  AllPortsSameDT=off  OutDataTypeStr=boolean
  OR14 : Logic  Operator=OR  AllPortsSameDT=off  OutDataTypeStr=boolean
  OR15 : Logic  Operator=OR  Inputs=5  AllPortsSameDT=off  OutDataTypeStr=boolean
  OUTPUT ONLY ON or READY : Subsystem
  Regen Level Switch : Stateflow chart  TreatAsAtomicUnit=on
  Regen Level Switch Botton : Subsystem
  Relational Operator3 : RelationalOperator  Operator=>  OutDataTypeStr=boolean  RndMeth=Simplest
  Relational Operator4 : RelationalOperator  Operator===  OutDataTypeStr=boolean  RndMeth=Simplest
  SR_Latch4 : hcu_lib/Basic_Blocks/SR_Latch
  Switch{13,15,17..18,20..24,27,29} (11 alike) : Switch  Criteria=u2 ~= 0
      Switch13 settings: AttributesFormatString=%<Criteria>
      Switch17 settings: AttributesFormatString=%<Criteria>
      Switch18 settings: AttributesFormatString=%<Criteria>
      Switch20 settings: AttributesFormatString=%<Criteria>
      Switch21 settings: AttributesFormatString=%<Criteria>
      Switch22 settings: AttributesFormatString=%<Criteria>
      Switch23 settings: AttributesFormatString=%<Criteria>
      Switch24 settings: AttributesFormatString=%<Criteria>
      Switch27 settings: AttributesFormatString=%<Criteria>
      Switch29 settings: AttributesFormatString=%<Criteria>
  Switch28 : Switch  Criteria=u2 > Threshold
      settings: AttributesFormatString=%<Criteria>
  SWC_RegenUp : Outport
  SWC_RegenDown : Outport  Port=2
  VTQD_FDCVCURegenMode_enum : Outport  Port=3
  VTQD_SaveRegenMode_enum : Outport  Port=4
  VTQD_TrailerDisOPDSta_flg : Outport  Port=5
  wires:
  Constant88/1 -> Switch22/1
  [VINP_SmartEcoModeSW_flg] -> Detect Increase/1
  [VINP_IVISnowModeCmd_flg] -> Regen Level Switch/5(VINP_IVISnowModeCmd_flg)
  Constant102/1 -> Switch27/3
  Switch20/1 -> [VTQD_FDCVCURegenMode_enum]  "VTQD_FDCVCURegenMode_enum"
  OUTPUT ONLY ON or READY/2(SWC_RegenDown) -> [SWC_RegenDown], Regen Level Switch Botton/3(SWC_RegenDown)
  [VINP_ADASACCSta_enum] -> OUTPUT ONLY ON or READY/4(VINP_ADASACCSta_enum)
  [VBCM_BrakeLamp_flg] -> OUTPUT ONLY ON or READY/6(VBCM_BrakeLamp_flg)
  [VTQD_SWCRegenUpSta_flg] -> OUTPUT ONLY ON or READY/2(VTQD_SWCRegenUpSta_flg)
  [VINP_VehSpeed_kph] -> OUTPUT ONLY ON or READY/7(VINP_VehSpeed_kph)
  [VVMC_CCCtrlSta_enum] -> OUTPUT ONLY ON or READY/5(VVMC_CCCtrlSta_enum)
  Delay6/1 -> Equal41/1
  [VDDM_SWCRegenUpSta_flg] -> Switch17/2
  AND8/1 -> DelayEnable/1
  KTQD_ICERoadDisTemp_C KTQD_ICERoadTemp_C/1 -> NOT1/1
  Switch22/1 -> [VTQD_SaveRegenMode_enum]  "VTQD_SaveRegenMode_enum"
  NOT1/1 -> AND8/2  "VTQD_ICERoad_flg"
  Max1/1 -> Relational Operator3/1
  [VTQD_RRSlideRate_pct] -> Add2/2
  Abs3/1 -> Max1/1
  [VTQD_LFSlideRate_pct] -> Add1/1
  " "/1 -> Switch20/1
  [VTQD_ActRgnUserSet_enum] -> Regen Level Switch/8(VTQD_ActRgnUserSet_enum)
  [VTQD_RegenMode_enum] -> Delay6/1
  Constant100/1 -> Switch18/1
  [VTQD_SCPSWCRegenUp_flg] -> Switch17/3
  Add2/1 -> Abs4/1
  Constant99/1 -> Switch17/1
  Constant95/1 -> Equal41/2
  Abs4/1 -> Max1/2
  [VTQD_BCMRgnUserEn_flg] -> Regen Level Switch/7(VTQD_BCMRgnUserEn_flg)
  Equal42/1 -> SR_Latch4/2
  [VBCM_UserNow_enum] -> Regen Level Switch/9(VBCM_BCMUserNowSetting_enum)
  Constant87/1 -> Switch22/2
  Constant110/1 -> DelayEnable/2
  [VTQD_ReadRegenMode_enum] -> Regen Level Switch/3(VTQD_ReadRegenMode_enum)
  [VTQD_RFSlideRate_pct] -> Add1/2
  Regen Level Switch Botton/1(VTQD_RegenSWSta_enum) -> [VTQD_RegenSWSta_enum]  "VTQD_RegenSWSta_enum"
  [VDDM_SWCRegenDownSta_flg] -> Switch18/2
  Constant115/1 -> [VDDM_SWCRegenDownSta_flg]  "VDDM_SWCRegenDownSta_flg"
  Detect Increase/1 -> Regen Level Switch/4(VINP_SmartEcoModeSW_flg)
  [VTQD_SCPSWCRegenDown_flg] -> Switch18/3
  DelayEnable/1 -> SR_Latch4/1
  Switch17/1 -> [VTQD_SWCRegenUpSta_flg]  "VTQD_SWCRegenUpSta_flg"
  [VTQD_LRSlideRate_pct] -> Add2/1
  [VTQD_SWCRegenDownSta_flg] -> OUTPUT ONLY ON or READY/3(VTQD_SWCRegenDownSta_flg)
  [VTQD_GearActualPosn_enum] -> Equal42/1
  Constant92/1 -> Relational Operator3/2
  "  "/1 -> Switch20/2
  Switch18/1 -> [VTQD_SWCRegenDownSta_flg]  "VTQD_SWCRegenDownSta_flg"
  [VPMM_PowerSta_enum] -> OUTPUT ONLY ON or READY/1(VPMM_PowerSta_enum)
  Constant111/1 -> Equal42/2
  Constant101/1 -> Switch27/2
  SR_Latch4/1 -> [VTQD_OPDModeDis_flg]  "VTQD_OPDModeDis_flg"
  Constant114/1 -> [VDDM_SWCRegenUpSta_flg]  "VDDM_SWCRegenUpSta_flg"
  Constant94/1 -> KTQD_ICERoadDisTemp_C KTQD_ICERoadTemp_C/1  "VTQD_OutSideTemp_C"
  Add1/1 -> Abs3/1
  [VTQD_TrailerMode_flg] -> Regen Level Switch/6(VTQD_TrailerMode_flg)
  Equal41/1 -> AND8/3
  [VPMM_PowerSta_enum] -> Regen Level Switch/1(VPMM_PowerSta_enum)
  [VINP_FlashRegenMode_enum] -> Switch27/1
  [task_time_s] -> Regen Level Switch Botton/1(task_time_s)
  [task_time_s] -> DelayEnable/3
  [VTQD_OPDModeDis_flg] -> Regen Level Switch/10(VTQD_OPDModeDis_flg)
  Relational Operator3/1 -> AND8/1
  BSCPIn_outputs/1 -> Bus Selector/1
  Bus Selector/2 -> [VINP_FlashRegenMode_enum]  "<VINP_FlashRegenMode_enum>"
  Bus Selector/6 -> [VBCM_BrakeLamp_flg]  "<VBCM_BrakeLamp_flg>"
  Bus Selector/9 -> [VINP_IVISnowModeCmd_flg]  "<VINP_IVISnowModeCmd_flg>"
  Bus Selector/10 -> [VBCM_UserNow_enum]  "<VBCM_UserNow_enum>"
  Bus Selector/11 -> [VINP_IVITrailerModeSWSta_flg]  "<VINP_IVITrailerModeSWSta_flg>"
  Bus Selector/12 -> [VINP_VehicleType_enum]  "<VINP_VehicleType_enum>"
  Bus Selector/13 -> [VBCM_RegenModeUserSetting_enum]  "<VBCM_RegenModeUserSetting_enum>"
  BSignalConvert_outputs/1 -> Bus Selector2/1
  Bus Selector2/1 -> [VTQD_RegenMode_enum]  "<VTQD_RegenMode_enum>"
  OUTPUT ONLY ON or READY/1(SWC_RegenUp) -> Regen Level Switch Botton/2(SWC_RegenUp), [SWC_RegenUp]
  [SWC_RegenUp] -> SWC_RegenUp/1
  [SWC_RegenDown] -> SWC_RegenDown/1
  [VTQD_FDCVCURegenMode_enum] -> VTQD_FDCVCURegenMode_enum/1
  [VTQD_SaveRegenMode_enum] -> VTQD_SaveRegenMode_enum/1
  [VTQD_TrailerDisOPDSta_flg] -> VTQD_TrailerDisOPDSta_flg/1
  VTQD_LFSlideRate_pct/1 -> [VTQD_LFSlideRate_pct]
  VTQD_RRSlideRate_pct/1 -> [VTQD_RRSlideRate_pct]
  VTQD_LRSlideRate_pct/1 -> [VTQD_LRSlideRate_pct]
  VTQD_RFSlideRate_pct/1 -> [VTQD_RFSlideRate_pct]
  VTQD_GearActualPosn_enum/1 -> [VTQD_GearActualPosn_enum]
  Constant118/1 -> Equal46/2
  [VBCM_UserNow_enum] -> Equal58/1
  Constant143/1 -> Equal59/2
  Detect Change3/1 -> AND24/5
  Equal55/1 -> OR14/2
  Equal58/1 -> AND24/4
  Equal56/1 -> AND24/2
  Constant112/1 -> Equal44/2
  Equal45/1 -> AND24/8
  Constant138/1 -> Equal54/2
  Constant135/1 -> Switch28/2
  [VINP_VehicleType_enum] -> Equal45/1
  [VINP_VehicleType_enum] -> Equal47/1
  Equal57/1 -> AND24/3
  Constant141/1 -> Equal57/2
  Equal59/1 -> OR15/1
  Constant136/1 -> Switch28/1
  Switch29/1 -> [VTQD_ActRgnUserSet_enum]  "VTQD_ActRgnUserSet_enum"
  [VBCM_RegenModeUserSetting_enum] -> Switch29/3
  [VINP_IVITrailerModeSWSta_flg] -> Switch28/3
  Relational Operator4/1 -> AND23/2
  Switch28/1 -> [VTQD_TrailerMode_flg]  "VTQD_TrailerMode_flg"
  [VPMM_PowerSta_enum] -> Equal54/1
  [VBCM_RegenModeUserSetting_enum] -> Equal59/1
  [VPMM_PowerSta_enum] -> Equal55/1
  [VINP_VehicleType_enum] -> Equal43/1
  [VINP_VehicleType_enum] -> Equal44/1
  [VBCM_UserNow_enum] -> Detect Change3/1
  [VTQD_RegenSWSta_enum] -> Relational Operator4/1
  [VINP_VehicleType_enum] -> Equal46/1
  Constant139/1 -> Equal55/2
  Equal44/1 -> AND24/7
  Equal43/1 -> AND24/6
  [VTQD_ReadRegenMode_enum] -> Switch29/1
  OR15/1 -> Switch29/2
  Constant142/1 -> Equal58/2
  Constant137/1 -> Relational Operator4/2
  Equal54/1 -> OR14/1
  [VTQD_TrailerMode_flg] -> AND23/1
  Constant113/1 -> Equal45/2
  OR14/1 -> AND24/1
  Equal46/1 -> OR15/3
  [VBCM_UserNow_enum] -> Equal56/1
  Equal48/1 -> OR15/5
  AND23/1 -> [VTQD_TrailerDisOPDSta_flg]  "VTQD_TrailerDisOPDSta_flg"
  [VBCM_UserNow_enum] -> Equal57/1
  Equal47/1 -> OR15/4
  Equal60/1 -> OR15/2
  Constant91/1 -> Equal43/2
  Constant140/1 -> Equal56/2
  Constant144/1 -> Equal60/2
  AND24/1 -> [VTQD_BCMRgnUserEn_flg]  "VTQD_BCMRgnUserEn_flg"
  [VBCM_RegenModeUserSetting_enum] -> Equal60/1
  [VINP_VehicleType_enum] -> Equal48/1
  Constant117/1 -> Equal48/2
  Constant116/1 -> Equal47/2
  Bus Selector/1 -> [task_time_s]  "<task_time_s>"
  Bus Selector/3 -> [VPMM_PowerSta_enum]  "<VPMM_PowerSta_enum>"
  Bus Selector/4 -> [VINP_ADASACCSta_enum]  "<VINP_ADASACCSta_enum>"
  Bus Selector/5 -> [VVMC_CCCtrlSta_enum]  "<VVMC_CCCtrlSta_enum>"
  Bus Selector/7 -> [VINP_VehSpeed_kph]  "<VINP_VehSpeed_kph>"
  Bus Selector/8 -> [VINP_SmartEcoModeSW_flg]  "<VINP_SmartEcoModeSW_flg>"
  [VTQD_RegenSWSta_enum] -> Regen Level Switch/2(VTQD_RegenSWSta_enum)
  Bus Selector2/2 -> [VTQD_SCPSWCRegenUp_flg]  "<VTQD_SCPSWCRegenUp_flg>"
  Bus Selector2/3 -> [VTQD_SCPSWCRegenDown_flg]  "<VTQD_SCPSWCRegenDown_flg>"
  AND10/1 -> Switch15/2
  Switch15/1 -> Switch13/1
  Delay1/1 -> Switch15/1
  [VTQD_SaveRegenMode_enum] -> Delay9/1
  Detect Increase1/1 -> Latch/1
  Switch13/1 -> [VTQD_ReadRegenMode_enum]  "VTQD_ReadRegenMode_enum"
  Data Type Conversion7/1 -> Switch13/2
  Delay9/1 -> Detect Change1/1
  Equal2/1 -> AND10/1
  Detect Change1/1 -> AND10/2
  [VTQD_ReadRegenMode_enum] -> Delay5/1
  [VTQD_SaveRegenMode_enum] -> Delay1/1
  Constant1/1 -> Equal1/2
  Constant2/1 -> Equal2/2
  Delay7/1 -> Equal2/1
  [VPMM_SysPowerMode_enum] -> Equal1/1
  Latch/1 -> Data Type Conversion7/1
  Equal1/1 -> Detect Increase1/1
  [VTQD_SaveRegenMode_enum] -> Delay7/1
  Delay5/1 -> Switch15/3
  Switch27/1 -> Switch13/3
  Bus Selector/14 -> [VPMM_SysPowerMode_enum]  "<VPMM_SysPowerMode_enum>"
  Bus Selector/15 -> [VINP_DIDNVHPedalLim_flg]  "<VINP_DIDNVHPedalLim_flg>"
  [VINP_DIDNVHPedalLim_flg] -> Regen Level Switch Botton/4(VINP_DIDNVHPedalLim_flg)
  Constant3/1 -> Switch21/1
  AND11/1 -> Switch21/2  "VTQD_DOAOPDReqSW_flg"
  Switch21/1 -> Switch23/3
  Constant119/1 -> Switch23/1
  Regen Level Switch/1(VTQD_RegenMode_enum) -> Switch21/3
  [VINP_DIDNVHPedalLim_flg] -> Switch23/2
  [VTQD_DOALatchReq_flg] -> AND11/1
  Constant4/1 -> AND11/2
  Switch23/1 -> Switch20/3
  [VINP_DIDNVHPedalLim_flg] -> Switch24/2
  Constant120/1 -> Switch24/1
  Regen Level Switch/2(VTQD_SaveRegenMode_enum) -> Switch24/3
  Switch24/1 -> Switch22/3
  VTQD_DOALatchReq_flg/1 -> [VTQD_DOALatchReq_flg]
